simulink library "ddm"  (R2021b)
settings: Solver=VariableStepAuto  StartTime=0.0  StopTime=10.0  RelTol=1e-3
undefined symbols (not defined in the file or in its folder): ADDM_FrTMTqDev_X_Nm, ADDM_RrTMTqDev_X_Nm, ENUM_ADASACCSTA_ERROR, ENUM_ADASACCSTA_OFF, ENUM_ADASACCSTA_STANDBY, ENUM_ALLOWMOV_ALLOWREADY, ENUM_APS, ENUM_BRKSTA_ERROR, ENUM_BRKSTA_OFF, ENUM_BRKSTA_ON, ENUM_BRKSW_INVALID, ENUM_BRKSW_OFF, ENUM_BRKSW_ON, ENUM_CHGPREACTERRSTA_OBCPRE, ENUM_DCDCFAULTSTA_ANYFAULTLV1, ENUM_DCDCFAULTSTA_ANYFAULTLV2, ENUM_DRIVETRAIN_AWD, ENUM_DRIVETRAIN_FWD, ENUM_DRIVETRAIN_RWD, ENUM_EDUDRTSTA_NORMAL, ENUM_EPBSTA_APPLIED, ENUM_EPBSTA_RELEASED, ENUM_GEARACTUALPOSN_INVALID, ENUM_GEARACTUALPOSN_P, ENUM_HVBATTREADYPRE_READY, ENUM_MCUWARN_LV0, ENUM_MCUWARN_LV1, ENUM_MCUWARN_LV2, ENUM_MCUWARN_LV3, ENUM_MCUWARN_NOERROR, ENUM_OBCFAULTSTA_ANYFAULT, ENUM_PAS_R2F2, ENUM_PDFAULT_BATTPDFAIL, ENUM_PDFAULT_DCDCDISABLE, ENUM_PDFAULT_MCUDISABLE, ENUM_PDFAULT_MCUDISCHRG, ENUM_POWERSTA_OFF, ENUM_POWERSTA_ON, ENUM_POWERSTA_READY, ENUM_POWERSTA_STANDBY, ENUM_PRESSINDI_LOW, ENUM_PUFAULT_BATTUPFAIL, ENUM_PUFAULT_DCDCENABLEFAIL, ENUM_PUFAULT_PRECHRGCHKFAIL, ENUM_PUFAULT_SAFETYCHKFAIL, ENUM_PUSTATE_COMPLETED, ENUM_PWRSTASW_OFF, ENUM_PWRSTASW_OFFA, ENUM_PWRSTASW_OFFCHVCHRG, ENUM_PWRSTASW_OFFCLVCHRG, ENUM_PWRSTASW_ON, ENUM_PWRSTASW_ONHVCHRG, ENUM_PWRSTASW_READY, ENUM_PWRSTASW_STANDBY, ENUM_SHIFTCOMMAND_P, ENUM_SHIFTERERRSTA_PBUTTONFAILURE, ENUM_VEHMALFUNLV_2ND, ENUM_VEHMALFUNLV_3RD, ENUM_VEHMALFUNLV_4TH, ENUM_VEHMALFUNLV_NORMAL ... (+459)
libraries: hcu_lib x521, $bdroot x5, simulink x3
(part 11 of 25)

== system ddm/DDM/DDM/TPM/RFWheelTmpHigh ==
  note: Diagnostics and Fault Handling
  note: Release Condition After Decision
  note: Test Pass Criteria
  note: Test Detection Criteria
  task_time_s : Inport
  VPMM_PowerSta_enum : Inport  Port=2
  DTC_clear_request : Inport  Port=3
  VTPM_RFWheelTmpHigh_flg : Inport  Port=4
  Constant : Constant  Value=KDDM_RFWheelTmpHighDTC_cnt
  Constant1 : Constant  Value=KDDM_RFWheelTmpHighDTC_cnt
  Constant10 : Constant  Value=ENUM_POWERSTA_OFF
  Constant11 : Constant  Value=KDDM_RFWheelTmpHighPassSW_flg
  Constant12 : Constant  Value=FALSE
  Constant13 : Constant  Value=KDDM_RFWheelTmpHighCFSSW_flg
  Constant14 : Constant  Value=KDDM_RFWheelTmpHighDFSSW_flg
  Constant15 : Constant  Value=KDDM_RFWheelTmpHighPassTO_s
  Constant2 : Constant  Value=ENUM_POWERSTA_READY
  Constant24 : Constant  Value=TRUE
  Constant25 : Constant  Value=FALSE
  Constant3 : Constant  Value=ENUM_POWERSTA_ON
  Constant4 : Constant  Value=FALSE
  Constant46 : Constant  Value=KDDM_RFWheelTmpHighDetSW_flg
  Constant5 : Constant  Value=ENUM_POWERSTA_READY
  Constant6 : Constant  Value=KDDM_RFWheelTmpHighDetTO_s
  Constant7 : Constant  Value=ENUM_POWERSTA_ON
  Constant8 : Constant  Value=TRUE
  Constant9 : Constant  Value=KDDM_RFWheelTmpHighPassTO_s
  DTC_Couter : hcu_lib/Basic_Blocks/DTC_Couter
  DTC_Info : hcu_lib/Basic_Blocks/DTC_Info
  Data Type Conversion1 : DataTypeConversion  OutDataTypeStr=uint8
  Equal{1..5} (5 alike) : RelationalOperator  Operator===  OutDataTypeStr=boolean  RndMeth=Simplest
  Equal6 : RelationalOperator  OutDataTypeStr=boolean  RndMeth=Simplest
  Logical Operator{1,4..5,7..8} (5 alike) : Logic  Operator=OR  AllPortsSameDT=off  OutDataTypeStr=boolean
  Logical Operator12 : Logic  AllPortsSameDT=off  OutDataTypeStr=boolean
  Logical Operator15 : Logic  AllPortsSameDT=off  OutDataTypeStr=boolean
  Logical Operator18 : Logic  AllPortsSameDT=off  OutDataTypeStr=boolean
  Logical Operator19 : Logic  Inputs=3  AllPortsSameDT=off  OutDataTypeStr=boolean
  Logical Operator2 : Logic  Operator=NOT  AllPortsSameDT=off  OutDataTypeStr=boolean
  Logical Operator3 : Logic  Operator=OR  Inputs=3  AllPortsSameDT=off  OutDataTypeStr=boolean
  Logical Operator6 : Logic  Operator=NOT  AllPortsSameDT=off  OutDataTypeStr=boolean
  Relay : Relay  OnSwitchValue=ONE_INT  OffSwitchValue=ZERO_INT
  SR_Latch1 : Subsystem  mask(SR_Latch){}
      mask help: SR latch function.
  SR_Latch3 : hcu_lib/Basic_Blocks/SR_Latch
  SR_Latch4 : hcu_lib/Basic_Blocks/SR_Latch
  Switch{2..4,6} (4 alike) : Switch  Criteria=u2 ~= 0
  Test Detection Criteria : hcu_lib/Basic_Blocks/Test Detection Criteria
  Timer1 : hcu_lib/Basic_Blocks/Timer
  VDDM_RFWheelTmpHighDTC_raw32 : Outport
  wires:
  Logical Operator6/1 -> Timer1/1
  Constant15/1 -> Timer1/4
  Timer1/1 -> Equal6/1
  [task_time_s] -> Timer1/3
  [VDDM_RFWheelTmpHighChk_flg] -> SR_Latch1/2(reset)
  SR_Latch1/1(latched) -> [VDDM_RFWheelTmpHighPass_flg]
  Constant9/1 -> Equal6/2
  Equal6/1 -> SR_Latch1/1(set)
  Switch4/1 -> Logical Operator6/1, Timer1/2
  Switch6/1 -> Test Detection Criteria/1
  Constant12/1 -> Switch6/1
  [DTC_clear_request] -> Switch6/2
  Switch3/1 -> Switch6/3, [VDDM_RFWheelTmpHighChk_flg]
  VTPM_RFWheelTmpHigh_flg/1 -> [VTPM_RFWheelTmpHigh_flg]
  Logical Operator4/1 -> Switch4/2
  Equal3/1 -> Logical Operator4/1
  [VPMM_PowerSta_enum] -> Equal2/1
  Constant3/1 -> Equal3/2
  Constant2/1 -> Equal2/2
  Constant8/1 -> Switch4/3
  Equal2/1 -> Logical Operator4/2
  [VPMM_PowerSta_enum] -> Equal3/1
  [task_time_s] -> Test Detection Criteria/2
  Constant/1 -> Test Detection Criteria/3
  Constant6/1 -> Test Detection Criteria/4
  [VPMM_PowerSta_enum] -> Equal5/1
  Equal1/1 -> Logical Operator1/2
  Equal5/1 -> Logical Operator1/1
  Logical Operator1/1 -> Switch3/2
  Constant7/1 -> Equal5/2
  Constant5/1 -> Equal1/2
  Constant4/1 -> Switch3/3
  [VPMM_PowerSta_enum] -> Equal1/1
  [DTC_clear_request] -> DTC_Info/4
  [VDDM_RFWheelTmpHighPass_flg] -> DTC_Info/2
  [VDDM_RFWheelTmpHighDet_flg] -> DTC_Info/1
  Test Detection Criteria/1 -> [VDDM_RFWheelTmpHighDet_flg]  "VDDM_RFWheelTmpHighDet_flg"
  DTC_Info/1 -> VDDM_RFWheelTmpHighDTC_raw32/1  "VDDM_RFWheelTmpHighDTC_raw32"
  [VDDM_RFWheelTmpHighCFS_flg] -> DTC_Info/3
  [VPMM_PowerSta_enum] -> Equal4/1
  DTC_clear_request/1 -> [DTC_clear_request]
  [VDDM_RFWheelTmpHighCFSRls_flg] -> Logical Operator3/3
  Logical Operator18/1 -> [VDDM_RFWheelTmpHighCFS_flg]
  Constant14/1 -> Logical Operator12/1
  SR_Latch3/1 -> Logical Operator12/2
  Constant13/1 -> Logical Operator18/2
  Logical Operator12/1 -> [VDDM_RFWheelTmpHighDFS_flg]
  SR_Latch4/1 -> Logical Operator18/1
  [VDDM_RFWheelTmpHighCFSRls_flg] -> Logical Operator5/1
  [VDDM_RFWheelTmpHighPass_flg] -> Logical Operator3/2
  DTC_Couter/1 -> SR_Latch4/1
  Data Type Conversion1/1 -> [VDDM_RFWheelTmpHighDTC_cnt]  "VDDM_RFWheelTmpHighDTC_cnt"
  Constant46/1 -> Logical Operator19/2
  Logical Operator19/1 -> DTC_Couter/1
  Constant11/1 -> Logical Operator15/2
  Logical Operator15/1 -> DTC_Couter/2
  Constant1/1 -> DTC_Couter/3
  DTC_Couter/2 -> Data Type Conversion1/1
  Relay/1 -> SR_Latch3/1
  [VDDM_RFWheelTmpHighDet_flg] -> Logical Operator19/1
  Logical Operator3/1 -> Logical Operator15/1
  [VDDM_RFWheelTmpHighDTC_cnt] -> Relay/1
  Equal4/1 -> Logical Operator8/1
  Constant10/1 -> Equal4/2
  Constant24/1 -> Switch2/1
  [DTC_clear_request] -> Logical Operator8/2
  Switch2/1 -> [VDDM_RFWheelTmpHighCFSRls_flg]
  Constant25/1 -> Switch2/3
  Logical Operator8/1 -> Switch2/2
  VPMM_PowerSta_enum/1 -> [VPMM_PowerSta_enum]
  task_time_s/1 -> [task_time_s]
  [VTPM_RFWheelTmpHigh_flg] -> Switch3/1
  [VTPM_RFWheelTmpHigh_flg] -> Switch4/1
  Logical Operator2/1 -> Logical Operator19/3
  [DTC_clear_request] -> Logical Operator3/1, Logical Operator2/1
  [DTC_clear_request] -> Logical Operator5/2
  Logical Operator5/1 -> SR_Latch4/2
  [VDDM_RFWheelTmpHighCFS_flg] -> Logical Operator7/1
  [DTC_clear_request] -> Logical Operator7/2
  Logical Operator7/1 -> SR_Latch3/2

== system ddm/DDM/DDM/TPM/RRBatwarn ==
  note: Diagnostics and Fault Handling
  note: Release Condition After Decision
  note: Test Pass Criteria
  note: Test Detection Criteria
  task_time_s : Inport
  VPMM_PowerSta_enum : Inport  Port=2
  DTC_clear_request : Inport  Port=3
  VTPM_RRBatwarn_flg : Inport  Port=4
  Constant : Constant  Value=KDDM_RRBatwarnDTC_cnt
  Constant1 : Constant  Value=KDDM_RRBatwarnDTC_cnt
  Constant10 : Constant  Value=ENUM_POWERSTA_OFF
  Constant11 : Constant  Value=KDDM_RRBatwarnPassSW_flg
  Constant12 : Constant  Value=FALSE
  Constant13 : Constant  Value=KDDM_RRBatwarnCFSSW_flg
  Constant14 : Constant  Value=KDDM_RRBatwarnDFSSW_flg
  Constant15 : Constant  Value=KDDM_RRBatwarnDetTO_s
  Constant16 : Constant  Value=KDDM_RRBatwarnDetTO_s
  Constant2 : Constant  Value=ENUM_POWERSTA_READY
  Constant24 : Constant  Value=TRUE
  Constant25 : Constant  Value=FALSE
  Constant3 : Constant  Value=ENUM_POWERSTA_ON
  Constant4 : Constant  Value=FALSE
  Constant46 : Constant  Value=KDDM_RRBatwarnDetSW_flg
  Constant5 : Constant  Value=ENUM_POWERSTA_READY
  Constant6 : Constant  Value=KDDM_RRBatwarnDetTO_s
  Constant7 : Constant  Value=ENUM_POWERSTA_ON
  Constant8 : Constant  Value=TRUE
  DTC_Couter : hcu_lib/Basic_Blocks/DTC_Couter
  DTC_Info : hcu_lib/Basic_Blocks/DTC_Info
  Data Type Conversion1 : DataTypeConversion  OutDataTypeStr=uint8
  Equal{1..5} (5 alike) : RelationalOperator  Operator===  OutDataTypeStr=boolean  RndMeth=Simplest
  Equal6 : RelationalOperator  OutDataTypeStr=boolean  RndMeth=Simplest
  Logical Operator1 : Logic  Operator=OR  AllPortsSameDT=off  OutDataTypeStr=boolean
  Logical Operator12 : Logic  AllPortsSameDT=off  OutDataTypeStr=boolean
  Logical Operator15 : Logic  AllPortsSameDT=off  OutDataTypeStr=boolean
  Logical Operator18 : Logic  AllPortsSameDT=off  OutDataTypeStr=boolean
  Logical Operator19 : Logic  Inputs=3  AllPortsSameDT=off  OutDataTypeStr=boolean
  Logical Operator2 : Logic  Operator=NOT  AllPortsSameDT=off  OutDataTypeStr=boolean
  Logical Operator3 : Logic  Operator=OR  Inputs=3  AllPortsSameDT=off  OutDataTypeStr=boolean
  Logical Operator4 : Logic  Operator=OR  AllPortsSameDT=off  OutDataTypeStr=boolean
  Logical Operator5 : Logic  Operator=OR  Inputs=2.  AllPortsSameDT=off  OutDataTypeStr=boolean
  Logical Operator6 : Logic  Operator=NOT  AllPortsSameDT=off  OutDataTypeStr=boolean
  Logical Operator7 : Logic  Operator=OR  Inputs=2.  AllPortsSameDT=off  OutDataTypeStr=boolean
  Logical Operator8 : Logic  Operator=OR  AllPortsSameDT=off  OutDataTypeStr=boolean
  Relay : Relay  OnSwitchValue=ONE_INT  OffSwitchValue=ZERO_INT
  SR_Latch1 : Subsystem  mask(SR_Latch){}
      mask help: SR latch function.
  SR_Latch3 : hcu_lib/Basic_Blocks/SR_Latch
  SR_Latch4 : hcu_lib/Basic_Blocks/SR_Latch
  Switch{2..4,6} (4 alike) : Switch  Criteria=u2 ~= 0
  Test Detection Criteria : hcu_lib/Basic_Blocks/Test Detection Criteria
  Timer1 : hcu_lib/Basic_Blocks/Timer
  VDDM_RRBatwarnDTC_raw32 : Outport
  wires:
  Switch6/1 -> Test Detection Criteria/1
  Constant12/1 -> Switch6/1
  [DTC_clear_request] -> Switch6/2
  Switch3/1 -> [VDDM_RRBatwarnChk_flg], Switch6/3
  VTPM_RRBatwarn_flg/1 -> [VTPM_RRBatwarn_flg]
  [VTPM_RRBatwarn_flg] -> Switch4/1
  Logical Operator4/1 -> Switch4/2
  Equal3/1 -> Logical Operator4/1
  [VPMM_PowerSta_enum] -> Equal2/1
  Constant7/1 -> Equal3/2
  Constant5/1 -> Equal2/2
  Constant8/1 -> Switch4/3
  Equal2/1 -> Logical Operator4/2
  [VPMM_PowerSta_enum] -> Equal3/1
  [VTPM_RRBatwarn_flg] -> Switch3/1
  [task_time_s] -> Test Detection Criteria/2
  Constant/1 -> Test Detection Criteria/3
  Constant6/1 -> Test Detection Criteria/4
  [VPMM_PowerSta_enum] -> Equal5/1
  Equal1/1 -> Logical Operator1/2
  Equal5/1 -> Logical Operator1/1
  Logical Operator1/1 -> Switch3/2
  Constant3/1 -> Equal5/2
  Constant2/1 -> Equal1/2
  Constant4/1 -> Switch3/3
  [VPMM_PowerSta_enum] -> Equal1/1
  [DTC_clear_request] -> DTC_Info/4
  [VDDM_RRBatwarnPass_flg] -> DTC_Info/2
  [VDDM_RRBatwarnDet_flg] -> DTC_Info/1
  Test Detection Criteria/1 -> [VDDM_RRBatwarnDet_flg]  "VDDM_RRBatwarnDet_flg"
  DTC_Info/1 -> VDDM_RRBatwarnDTC_raw32/1  "VDDM_RRBatwarnDTC_raw32"
  [VDDM_RRBatwarnCFS_flg] -> DTC_Info/3
  [VPMM_PowerSta_enum] -> Equal4/1
  DTC_clear_request/1 -> [DTC_clear_request]
  [VDDM_RRBatwarnCFSRls_flg] -> Logical Operator3/3
  Logical Operator18/1 -> [VDDM_RRBatwarnCFS_flg]
  Constant14/1 -> Logical Operator12/1
  SR_Latch3/1 -> Logical Operator12/2
  Constant13/1 -> Logical Operator18/2
  Logical Operator12/1 -> [VDDM_RRBatwarnDFS_flg]
  SR_Latch4/1 -> Logical Operator18/1
  [VDDM_RRBatwarnCFSRls_flg] -> Logical Operator5/1
  [VDDM_RRBatwarnPass_flg] -> Logical Operator3/2
  DTC_Couter/1 -> SR_Latch4/1
  Data Type Conversion1/1 -> [VDDM_RRBatwarnDTC_cnt]  "VDDM_RRBatwarnDTC_cnt"
  Constant46/1 -> Logical Operator19/2
  Logical Operator19/1 -> DTC_Couter/1
  Constant11/1 -> Logical Operator15/2
  Logical Operator15/1 -> DTC_Couter/2
  Constant1/1 -> DTC_Couter/3
  DTC_Couter/2 -> Data Type Conversion1/1
  Relay/1 -> SR_Latch3/1
  [VDDM_RRBatwarnDet_flg] -> Logical Operator19/1
  Logical Operator3/1 -> Logical Operator15/1
  [VDDM_RRBatwarnCFS_flg] -> Logical Operator7/1
  [VDDM_RRBatwarnDTC_cnt] -> Relay/1
  Equal4/1 -> Logical Operator8/1
  Constant10/1 -> Equal4/2
  Constant24/1 -> Switch2/1
  [DTC_clear_request] -> Logical Operator8/2
  Switch2/1 -> [VDDM_RRBatwarnCFSRls_flg]
  Constant25/1 -> Switch2/3
  Logical Operator8/1 -> Switch2/2
  VPMM_PowerSta_enum/1 -> [VPMM_PowerSta_enum]
  task_time_s/1 -> [task_time_s]
  Switch4/1 -> Timer1/2, Logical Operator6/1
  Equal6/1 -> SR_Latch1/1(set)
  [VDDM_RRBatwarnChk_flg] -> SR_Latch1/2(reset)
  Timer1/1 -> Equal6/1
  Constant16/1 -> Equal6/2
  SR_Latch1/1(latched) -> [VDDM_RRBatwarnPass_flg]
  [task_time_s] -> Timer1/3
  Logical Operator6/1 -> Timer1/1
  Constant15/1 -> Timer1/4
  Logical Operator2/1 -> Logical Operator19/3
  [DTC_clear_request] -> Logical Operator3/1, Logical Operator2/1
  Logical Operator5/1 -> SR_Latch4/2
  [DTC_clear_request] -> Logical Operator5/2
  Logical Operator7/1 -> SR_Latch3/2
  [DTC_clear_request] -> Logical Operator7/2

== system ddm/DDM/DDM/TPM/RRPressureLow ==
  note: Test Detection Criteria
  note: Test Pass Criteria
  note: Release Condition After Decision
  note: Diagnostics and Fault Handling
  task_time_s : Inport
  VPMM_PowerSta_enum : Inport  Port=2
  DTC_clear_request : Inport  Port=3
  VTPM_RRPressIndi_enum : Inport  Port=4
  Constant : Constant  Value=KDDM_RRPressIndiDTC_cnt
  Constant1 : Constant  Value=KDDM_RRPressIndiDTC_cnt
  Constant10 : Constant  Value=ENUM_POWERSTA_OFF
  Constant11 : Constant  Value=KDDM_RRPressIndiPassSW_flg
  Constant12 : Constant  Value=FALSE
  Constant13 : Constant  Value=KDDM_RRPressIndiCFSSW_flg
  Constant14 : Constant  Value=KDDM_RRPressIndiDFSSW_flg
  Constant15 : Constant  Value=KDDM_RRPressIndiPassTO_s
  Constant16 : Constant  Value=ENUM_PRESSINDI_LOW
  Constant17 : Constant  Value=ENUM_PRESSINDI_LOW
  Constant2 : Constant  Value=ENUM_POWERSTA_READY
  Constant24 : Constant  Value=TRUE
  Constant25 : Constant  Value=FALSE
  Constant3 : Constant  Value=ENUM_POWERSTA_ON
  Constant4 : Constant  Value=FALSE
  Constant46 : Constant  Value=KDDM_RRPressIndiDetSW_flg
  Constant5 : Constant  Value=ENUM_POWERSTA_READY
  Constant6 : Constant  Value=KDDM_RRPressIndiDetTO_s
  Constant7 : Constant  Value=ENUM_POWERSTA_ON
  Constant8 : Constant  Value=TRUE
  Constant9 : Constant  Value=KDDM_RRPressIndiPassTO_s
  DTC_Couter : hcu_lib/Basic_Blocks/DTC_Couter
  DTC_Info : hcu_lib/Basic_Blocks/DTC_Info
  Data Type Conversion1 : DataTypeConversion  OutDataTypeStr=uint8
  Equal{1..5,7..8} (7 alike) : RelationalOperator  Operator===  OutDataTypeStr=boolean  RndMeth=Simplest
  Equal6 : RelationalOperator  OutDataTypeStr=boolean  RndMeth=Simplest
  Logical Operator{1,4..5,7..8} (5 alike) : Logic  Operator=OR  AllPortsSameDT=off  OutDataTypeStr=boolean
  Logical Operator12 : Logic  AllPortsSameDT=off  OutDataTypeStr=boolean
  Logical Operator15 : Logic  AllPortsSameDT=off  OutDataTypeStr=boolean
  Logical Operator18 : Logic  AllPortsSameDT=off  OutDataTypeStr=boolean
  Logical Operator19 : Logic  Inputs=3  AllPortsSameDT=off  OutDataTypeStr=boolean
  Logical Operator2 : Logic  Operator=NOT  AllPortsSameDT=off  OutDataTypeStr=boolean
  Logical Operator3 : Logic  Operator=OR  Inputs=3  AllPortsSameDT=off  OutDataTypeStr=boolean
  Logical Operator6 : Logic  Operator=NOT  AllPortsSameDT=off  OutDataTypeStr=boolean
  Relay : Relay  OnSwitchValue=ONE_INT  OffSwitchValue=ZERO_INT
  SR_Latch1 : Subsystem  mask(SR_Latch){}
      mask help: SR latch function.
  SR_Latch3 : hcu_lib/Basic_Blocks/SR_Latch
  SR_Latch4 : hcu_lib/Basic_Blocks/SR_Latch
  Switch{2..4,6} (4 alike) : Switch  Criteria=u2 ~= 0
  Test Detection Criteria : hcu_lib/Basic_Blocks/Test Detection Criteria
  Timer1 : hcu_lib/Basic_Blocks/Timer
  VDDM_RRPressIndiDTC_raw32 : Outport
  wires:
  [VTPM_RRPressIndi_enum] -> Equal8/1
  Constant17/1 -> Equal8/2
  Equal8/1 -> Switch4/1
  Constant16/1 -> Equal7/2
  Equal7/1 -> Switch3/1
  [VTPM_RRPressIndi_enum] -> Equal7/1
  task_time_s/1 -> [task_time_s]
  VPMM_PowerSta_enum/1 -> [VPMM_PowerSta_enum]
  Logical Operator8/1 -> Switch2/2
  Constant25/1 -> Switch2/3
  Switch2/1 -> [VDDM_RRPressIndiCFSRls_flg]
  [DTC_clear_request] -> Logical Operator8/2
  Constant24/1 -> Switch2/1
  Constant10/1 -> Equal4/2
  Equal4/1 -> Logical Operator8/1
  [VDDM_RRPressIndiDTC_cnt] -> Relay/1
  [VDDM_RRPressIndiCFS_flg] -> Logical Operator7/1
  Logical Operator3/1 -> Logical Operator15/1
  [VDDM_RRPressIndiDet_flg] -> Logical Operator19/1
  Relay/1 -> SR_Latch3/1
  Constant1/1 -> DTC_Couter/3
  Logical Operator15/1 -> DTC_Couter/2
  Constant11/1 -> Logical Operator15/2
  Logical Operator19/1 -> DTC_Couter/1
  Constant46/1 -> Logical Operator19/2
  DTC_Couter/1 -> SR_Latch4/1
  [VDDM_RRPressIndiPass_flg] -> Logical Operator3/2
  [VDDM_RRPressIndiCFSRls_flg] -> Logical Operator5/1
  SR_Latch4/1 -> Logical Operator18/1
  Logical Operator12/1 -> [VDDM_RRPressIndiDFS_flg]
  Constant13/1 -> Logical Operator18/2
  SR_Latch3/1 -> Logical Operator12/2
  Constant14/1 -> Logical Operator12/1
  Logical Operator18/1 -> [VDDM_RRPressIndiCFS_flg]
  [VDDM_RRPressIndiCFSRls_flg] -> Logical Operator3/3
  DTC_clear_request/1 -> [DTC_clear_request]
  [VPMM_PowerSta_enum] -> Equal4/1
  [VDDM_RRPressIndiCFS_flg] -> DTC_Info/3
  DTC_Info/1 -> VDDM_RRPressIndiDTC_raw32/1  "VDDM_RRPressIndiDTC_raw32"
  Test Detection Criteria/1 -> [VDDM_RRPressIndiDet_flg]  "VDDM_RRPressIndiDet_flg"
  [VDDM_RRPressIndiDet_flg] -> DTC_Info/1
  [VDDM_RRPressIndiPass_flg] -> DTC_Info/2
  [DTC_clear_request] -> DTC_Info/4
  [VPMM_PowerSta_enum] -> Equal1/1
  Constant4/1 -> Switch3/3
  Constant5/1 -> Equal1/2
  Constant7/1 -> Equal5/2
  Logical Operator1/1 -> Switch3/2
  Equal5/1 -> Logical Operator1/1
  Equal1/1 -> Logical Operator1/2
  [VPMM_PowerSta_enum] -> Equal5/1
  Constant6/1 -> Test Detection Criteria/4
  Constant/1 -> Test Detection Criteria/3
  [task_time_s] -> Test Detection Criteria/2
  [VPMM_PowerSta_enum] -> Equal3/1
  Equal2/1 -> Logical Operator4/2
  Constant8/1 -> Switch4/3
  Constant2/1 -> Equal2/2
  Constant3/1 -> Equal3/2
  [VPMM_PowerSta_enum] -> Equal2/1
  Equal3/1 -> Logical Operator4/1
  Logical Operator4/1 -> Switch4/2
  VTPM_RRPressIndi_enum/1 -> [VTPM_RRPressIndi_enum]
  Switch3/1 -> [VDDM_RRPressIndiChk_flg], Switch6/3
  [DTC_clear_request] -> Switch6/2
  Constant12/1 -> Switch6/1
  Switch6/1 -> Test Detection Criteria/1
  Switch4/1 -> Logical Operator6/1, Timer1/2
  Equal6/1 -> SR_Latch1/1(set)
  Constant9/1 -> Equal6/2
  SR_Latch1/1(latched) -> [VDDM_RRPressIndiPass_flg]
  [VDDM_RRPressIndiChk_flg] -> SR_Latch1/2(reset)
  [task_time_s] -> Timer1/3
  Timer1/1 -> Equal6/1
  Constant15/1 -> Timer1/4
  Logical Operator6/1 -> Timer1/1
  Data Type Conversion1/1 -> [VDDM_RRPressIndiDTC_cnt]  "VDDM_RRPressIndiDTC_cnt"
  DTC_Couter/2 -> Data Type Conversion1/1
  Logical Operator2/1 -> Logical Operator19/3
  [DTC_clear_request] -> Logical Operator3/1, Logical Operator2/1
  Logical Operator5/1 -> SR_Latch4/2
  [DTC_clear_request] -> Logical Operator5/2
  Logical Operator7/1 -> SR_Latch3/2
  [DTC_clear_request] -> Logical Operator7/2

== system ddm/DDM/DDM/TPM/RRSensorfail ==
  note: Test Detection Criteria
  note: Test Pass Criteria
  note: Release Condition After Decision
  note: Diagnostics and Fault Handling
  task_time_s : Inport
  VPMM_PowerSta_enum : Inport  Port=2
  DTC_clear_request : Inport  Port=3
  VTPM_RRSensorFail_flg : Inport  Port=4
  Constant : Constant  Value=KDDM_RRSensorFailDTC_cnt
  Constant1 : Constant  Value=KDDM_RRSensorFailDTC_cnt
  Constant10 : Constant  Value=ENUM_POWERSTA_OFF
  Constant11 : Constant  Value=KDDM_RRSensorFailPassSW_flg
  Constant12 : Constant  Value=FALSE
  Constant13 : Constant  Value=KDDM_RRSensorFailCFSSW_flg
  Constant14 : Constant  Value=KDDM_RRSensorFailDFSSW_flg
  Constant15 : Constant  Value=KDDM_RRSensorFailPassTO_s
  Constant2 : Constant  Value=ENUM_POWERSTA_READY
  Constant24 : Constant  Value=TRUE
  Constant25 : Constant  Value=FALSE
  Constant3 : Constant  Value=ENUM_POWERSTA_ON
  Constant4 : Constant  Value=FALSE
  Constant46 : Constant  Value=KDDM_RRSensorFailDetSW_flg
  Constant5 : Constant  Value=ENUM_POWERSTA_READY
  Constant6 : Constant  Value=KDDM_RRSensorFailDetTO_s
  Constant7 : Constant  Value=ENUM_POWERSTA_ON
  Constant8 : Constant  Value=TRUE
  Constant9 : Constant  Value=KDDM_RRSensorFailPassTO_s
  DTC_Couter : hcu_lib/Basic_Blocks/DTC_Couter
  DTC_Info : hcu_lib/Basic_Blocks/DTC_Info
  Data Type Conversion1 : DataTypeConversion  OutDataTypeStr=uint8
  Equal{1..5} (5 alike) : RelationalOperator  Operator===  OutDataTypeStr=boolean  RndMeth=Simplest
  Equal6 : RelationalOperator  OutDataTypeStr=boolean  RndMeth=Simplest
  Logical Operator{1..2,4,7..8} (5 alike) : Logic  Operator=OR  AllPortsSameDT=off  OutDataTypeStr=boolean
  Logical Operator12 : Logic  AllPortsSameDT=off  OutDataTypeStr=boolean
  Logical Operator15 : Logic  AllPortsSameDT=off  OutDataTypeStr=boolean
  Logical Operator18 : Logic  AllPortsSameDT=off  OutDataTypeStr=boolean
  Logical Operator19 : Logic  Inputs=3  AllPortsSameDT=off  OutDataTypeStr=boolean
  Logical Operator3 : Logic  Operator=OR  Inputs=3  AllPortsSameDT=off  OutDataTypeStr=boolean
  Logical Operator5 : Logic  Operator=NOT  AllPortsSameDT=off  OutDataTypeStr=boolean
  Logical Operator6 : Logic  Operator=NOT  AllPortsSameDT=off  OutDataTypeStr=boolean
  Relay : Relay  OnSwitchValue=ONE_INT  OffSwitchValue=ZERO_INT
  SR_Latch1 : Subsystem  mask(SR_Latch){}
      mask help: SR latch function.
  SR_Latch3 : hcu_lib/Basic_Blocks/SR_Latch
  SR_Latch4 : hcu_lib/Basic_Blocks/SR_Latch
  Switch{2..4,6} (4 alike) : Switch  Criteria=u2 ~= 0
  Test Detection Criteria : hcu_lib/Basic_Blocks/Test Detection Criteria
  Timer1 : hcu_lib/Basic_Blocks/Timer
  VDDM_RRSensorFailDTC_raw32 : Outport
  wires:
  [VTPM_RRSensorFail_flg] -> Switch4/1
  [VTPM_RRSensorFail_flg] -> Switch3/1
  task_time_s/1 -> [task_time_s]
  VPMM_PowerSta_enum/1 -> [VPMM_PowerSta_enum]
  Logical Operator8/1 -> Switch2/2
  Constant25/1 -> Switch2/3
  Switch2/1 -> [VDDM_RRSensorFailCFSRls_flg]
  [DTC_clear_request] -> Logical Operator8/2
  Constant24/1 -> Switch2/1
  Constant10/1 -> Equal4/2
  Equal4/1 -> Logical Operator8/1
  [VDDM_RRSensorFailDTC_cnt] -> Relay/1
  [VDDM_RRSensorFailCFS_flg] -> Logical Operator7/1
  Logical Operator3/1 -> Logical Operator15/1
  [VDDM_RRSensorFailDet_flg] -> Logical Operator19/1
  Relay/1 -> SR_Latch3/1
  DTC_Couter/2 -> Data Type Conversion1/1
  Constant1/1 -> DTC_Couter/3
  Logical Operator15/1 -> DTC_Couter/2
  Constant11/1 -> Logical Operator15/2
  Logical Operator19/1 -> DTC_Couter/1
  Constant46/1 -> Logical Operator19/2
  Data Type Conversion1/1 -> [VDDM_RRSensorFailDTC_cnt]  "VDDM_RRSensorFailDTC_cnt"
  DTC_Couter/1 -> SR_Latch4/1
  [VDDM_RRSensorFailPass_flg] -> Logical Operator3/2
  [VDDM_RRSensorFailCFSRls_flg] -> Logical Operator2/1
  SR_Latch4/1 -> Logical Operator18/1
  Logical Operator12/1 -> [VDDM_RRSensorFailDFS_flg]
  Constant13/1 -> Logical Operator18/2
  SR_Latch3/1 -> Logical Operator12/2
  Constant14/1 -> Logical Operator12/1
  Logical Operator18/1 -> [VDDM_RRSensorFailCFS_flg]
  [VDDM_RRSensorFailCFSRls_flg] -> Logical Operator3/3
  DTC_clear_request/1 -> [DTC_clear_request]
  [VPMM_PowerSta_enum] -> Equal4/1
  [VDDM_RRSensorFailCFS_flg] -> DTC_Info/3
  DTC_Info/1 -> VDDM_RRSensorFailDTC_raw32/1  "VDDM_RRSensorFailDTC_raw32"
  Test Detection Criteria/1 -> [VDDM_RRSensorFailDet_flg]  "VDDM_RRSensorFailDet_flg"
  [VDDM_RRSensorFailDet_flg] -> DTC_Info/1
  [VDDM_RRSensorFailPass_flg] -> DTC_Info/2
  [DTC_clear_request] -> DTC_Info/4
  [VPMM_PowerSta_enum] -> Equal1/1
  Constant4/1 -> Switch3/3
  Constant5/1 -> Equal1/2
  Constant7/1 -> Equal5/2
  Logical Operator1/1 -> Switch3/2
  Equal5/1 -> Logical Operator1/1
  Equal1/1 -> Logical Operator1/2
  [VPMM_PowerSta_enum] -> Equal5/1
  Constant6/1 -> Test Detection Criteria/4
  Constant/1 -> Test Detection Criteria/3
  [task_time_s] -> Test Detection Criteria/2
  [VPMM_PowerSta_enum] -> Equal3/1
  Equal2/1 -> Logical Operator4/2
  Constant8/1 -> Switch4/3
  Constant2/1 -> Equal2/2
  Constant3/1 -> Equal3/2
  [VPMM_PowerSta_enum] -> Equal2/1
  Equal3/1 -> Logical Operator4/1
  Logical Operator4/1 -> Switch4/2
  VTPM_RRSensorFail_flg/1 -> [VTPM_RRSensorFail_flg]
  Switch3/1 -> [VDDM_RRSensorFailChk_flg], Switch6/3
  [DTC_clear_request] -> Switch6/2
  Constant12/1 -> Switch6/1
  Switch6/1 -> Test Detection Criteria/1
  Switch4/1 -> Timer1/2, Logical Operator6/1
  Equal6/1 -> SR_Latch1/1(set)
  Constant9/1 -> Equal6/2
  SR_Latch1/1(latched) -> [VDDM_RRSensorFailPass_flg]
  [VDDM_RRSensorFailChk_flg] -> SR_Latch1/2(reset)
  [task_time_s] -> Timer1/3
  Timer1/1 -> Equal6/1
  Constant15/1 -> Timer1/4
  Logical Operator6/1 -> Timer1/1
  Logical Operator5/1 -> Logical Operator19/3
  [DTC_clear_request] -> Logical Operator3/1, Logical Operator5/1
  Logical Operator2/1 -> SR_Latch4/2
  [DTC_clear_request] -> Logical Operator2/2
  Logical Operator7/1 -> SR_Latch3/2
  [DTC_clear_request] -> Logical Operator7/2

== system ddm/DDM/DDM/TPM/RRWheelTmpHigh ==
  note: Diagnostics and Fault Handling
  note: Release Condition After Decision
  note: Test Pass Criteria
  note: Test Detection Criteria
  task_time_s : Inport
  VPMM_PowerSta_enum : Inport  Port=2
  DTC_clear_request : Inport  Port=3
  VTPM_RRWheelTmpHigh_flg : Inport  Port=4
  Constant : Constant  Value=KDDM_RRWheelTmpHighDTC_cnt
  Constant1 : Constant  Value=KDDM_RRWheelTmpHighDTC_cnt
  Constant10 : Constant  Value=ENUM_POWERSTA_OFF
  Constant11 : Constant  Value=KDDM_RRWheelTmpHighPassSW_flg
  Constant12 : Constant  Value=FALSE
  Constant13 : Constant  Value=KDDM_RRWheelTmpHighCFSSW_flg
  Constant14 : Constant  Value=KDDM_RRWheelTmpHighDFSSW_flg
  Constant15 : Constant  Value=KDDM_RRWheelTmpHighPassTO_s
  Constant2 : Constant  Value=ENUM_POWERSTA_READY
  Constant24 : Constant  Value=TRUE
  Constant25 : Constant  Value=FALSE
  Constant3 : Constant  Value=ENUM_POWERSTA_ON
  Constant4 : Constant  Value=FALSE
  Constant46 : Constant  Value=KDDM_RRWheelTmpHighDetSW_flg
  Constant5 : Constant  Value=ENUM_POWERSTA_READY
  Constant6 : Constant  Value=KDDM_RRWheelTmpHighDetTO_s
  Constant7 : Constant  Value=ENUM_POWERSTA_ON
  Constant8 : Constant  Value=TRUE
  Constant9 : Constant  Value=KDDM_RRWheelTmpHighPassTO_s
  DTC_Couter : hcu_lib/Basic_Blocks/DTC_Couter
  DTC_Info : hcu_lib/Basic_Blocks/DTC_Info
  Data Type Conversion1 : DataTypeConversion  OutDataTypeStr=uint8
  Equal{1..5} (5 alike) : RelationalOperator  Operator===  OutDataTypeStr=boolean  RndMeth=Simplest
  Equal6 : RelationalOperator  OutDataTypeStr=boolean  RndMeth=Simplest
  Logical Operator{1..2,4,7..8} (5 alike) : Logic  Operator=OR  AllPortsSameDT=off  OutDataTypeStr=boolean
  Logical Operator12 : Logic  AllPortsSameDT=off  OutDataTypeStr=boolean
  Logical Operator15 : Logic  AllPortsSameDT=off  OutDataTypeStr=boolean
  Logical Operator18 : Logic  AllPortsSameDT=off  OutDataTypeStr=boolean
  Logical Operator19 : Logic  Inputs=3  AllPortsSameDT=off  OutDataTypeStr=boolean
  Logical Operator3 : Logic  Operator=OR  Inputs=3  AllPortsSameDT=off  OutDataTypeStr=boolean
  Logical Operator5 : Logic  Operator=NOT  AllPortsSameDT=off  OutDataTypeStr=boolean
  Logical Operator6 : Logic  Operator=NOT  AllPortsSameDT=off  OutDataTypeStr=boolean
  Relay : Relay  OnSwitchValue=ONE_INT  OffSwitchValue=ZERO_INT
  SR_Latch1 : Subsystem  mask(SR_Latch){}
      mask help: SR latch function.
  SR_Latch3 : hcu_lib/Basic_Blocks/SR_Latch
  SR_Latch4 : hcu_lib/Basic_Blocks/SR_Latch
  Switch{2..4,6} (4 alike) : Switch  Criteria=u2 ~= 0
  Test Detection Criteria : hcu_lib/Basic_Blocks/Test Detection Criteria
  Timer1 : hcu_lib/Basic_Blocks/Timer
  VDDM_RRWheelTmpHighDTC_raw32 : Outport
  wires:
  Logical Operator6/1 -> Timer1/1
  Constant15/1 -> Timer1/4
  Timer1/1 -> Equal6/1
  [task_time_s] -> Timer1/3
  [VDDM_RRWheelTmpHighChk_flg] -> SR_Latch1/2(reset)
  SR_Latch1/1(latched) -> [VDDM_RRWheelTmpHighPass_flg]
  Constant9/1 -> Equal6/2
  Equal6/1 -> SR_Latch1/1(set)
  Switch4/1 -> Logical Operator6/1, Timer1/2
  Switch6/1 -> Test Detection Criteria/1
  Constant12/1 -> Switch6/1
  [DTC_clear_request] -> Switch6/2
  Switch3/1 -> Switch6/3, [VDDM_RRWheelTmpHighChk_flg]
  VTPM_RRWheelTmpHigh_flg/1 -> [VTPM_RRWheelTmpHigh_flg]
  Logical Operator4/1 -> Switch4/2
  Equal3/1 -> Logical Operator4/1
  [VPMM_PowerSta_enum] -> Equal2/1
  Constant3/1 -> Equal3/2
  Constant2/1 -> Equal2/2
  Constant8/1 -> Switch4/3
  Equal2/1 -> Logical Operator4/2
  [VPMM_PowerSta_enum] -> Equal3/1
  [task_time_s] -> Test Detection Criteria/2
  Constant/1 -> Test Detection Criteria/3
  Constant6/1 -> Test Detection Criteria/4
  [VPMM_PowerSta_enum] -> Equal5/1
  Equal1/1 -> Logical Operator1/2
  Equal5/1 -> Logical Operator1/1
  Logical Operator1/1 -> Switch3/2
  Constant7/1 -> Equal5/2
  Constant5/1 -> Equal1/2
  Constant4/1 -> Switch3/3
  [VPMM_PowerSta_enum] -> Equal1/1
  [DTC_clear_request] -> DTC_Info/4
  [VDDM_RRWheelTmpHighPass_flg] -> DTC_Info/2
  [VDDM_RRWheelTmpHighDet_flg] -> DTC_Info/1
  Test Detection Criteria/1 -> [VDDM_RRWheelTmpHighDet_flg]  "VDDM_RRWheelTmpHighDet_flg"
  DTC_Info/1 -> VDDM_RRWheelTmpHighDTC_raw32/1  "VDDM_RRWheelTmpHighDTC_raw32"
  [VDDM_RRWheelTmpHighCFS_flg] -> DTC_Info/3
  [VPMM_PowerSta_enum] -> Equal4/1
  DTC_clear_request/1 -> [DTC_clear_request]
  [VDDM_RRWheelTmpHighCFSRls_flg] -> Logical Operator3/3
  Logical Operator18/1 -> [VDDM_RRWheelTmpHighCFS_flg]
  Constant14/1 -> Logical Operator12/1
  SR_Latch3/1 -> Logical Operator12/2
  Constant13/1 -> Logical Operator18/2
  Logical Operator12/1 -> [VDDM_RRWheelTmpHighDFS_flg]
  SR_Latch4/1 -> Logical Operator18/1
  [VDDM_RRWheelTmpHighCFSRls_flg] -> Logical Operator2/1
  [VDDM_RRWheelTmpHighPass_flg] -> Logical Operator3/2
  DTC_Couter/1 -> SR_Latch4/1
  Data Type Conversion1/1 -> [VDDM_RRWheelTmpHighDTC_cnt]  "VDDM_RRWheelTmpHighDTC_cnt"
  Constant46/1 -> Logical Operator19/2
  Logical Operator19/1 -> DTC_Couter/1
  Constant11/1 -> Logical Operator15/2
  Logical Operator15/1 -> DTC_Couter/2
  Constant1/1 -> DTC_Couter/3
  DTC_Couter/2 -> Data Type Conversion1/1
  Relay/1 -> SR_Latch3/1
  [VDDM_RRWheelTmpHighDet_flg] -> Logical Operator19/1
  Logical Operator3/1 -> Logical Operator15/1
  [VDDM_RRWheelTmpHighCFS_flg] -> Logical Operator7/1
  [VDDM_RRWheelTmpHighDTC_cnt] -> Relay/1
  Equal4/1 -> Logical Operator8/1
  Constant10/1 -> Equal4/2
  Constant24/1 -> Switch2/1
  [DTC_clear_request] -> Logical Operator8/2
  Switch2/1 -> [VDDM_RRWheelTmpHighCFSRls_flg]
  Constant25/1 -> Switch2/3
  Logical Operator8/1 -> Switch2/2
  VPMM_PowerSta_enum/1 -> [VPMM_PowerSta_enum]
  task_time_s/1 -> [task_time_s]
  [VTPM_RRWheelTmpHigh_flg] -> Switch3/1
  [VTPM_RRWheelTmpHigh_flg] -> Switch4/1
  Logical Operator5/1 -> Logical Operator19/3
  [DTC_clear_request] -> Logical Operator3/1, Logical Operator5/1
  Logical Operator2/1 -> SR_Latch4/2
  [DTC_clear_request] -> Logical Operator2/2
  Logical Operator7/1 -> SR_Latch3/2
  [DTC_clear_request] -> Logical Operator7/2
